simulink model "Copy_of_model_PID"  (R2015a)
settings: Solver=ode4  StartTime=0.0  StopTime=T_sim  FixedStep=0.01  RelTol=1e-3
values from neighbouring files (symbols this model uses):
  D1 = Nastawy(3)    [SzukanieNastaw.m]    (also in wskaznikJakosci.m = params(3))
  h0 = 5    [wskaznikJakosci.m]
  I1 = Nastawy(2)    [SzukanieNastaw.m]    (also in wskaznikJakosci.m = params(2))
  P1 = Nastawy(1)    [SzukanieNastaw.m]    (also in wskaznikJakosci.m = params(1))
  ref = 30    [wskaznikJakosci.m]
undefined symbols (not defined in the file or in its folder): pompaP1, sigbuilder_block, zaworC1, zaworC2, zaworP1
libraries: simulink x1
settings Model: Creator=konra  LastModifiedBy=konra

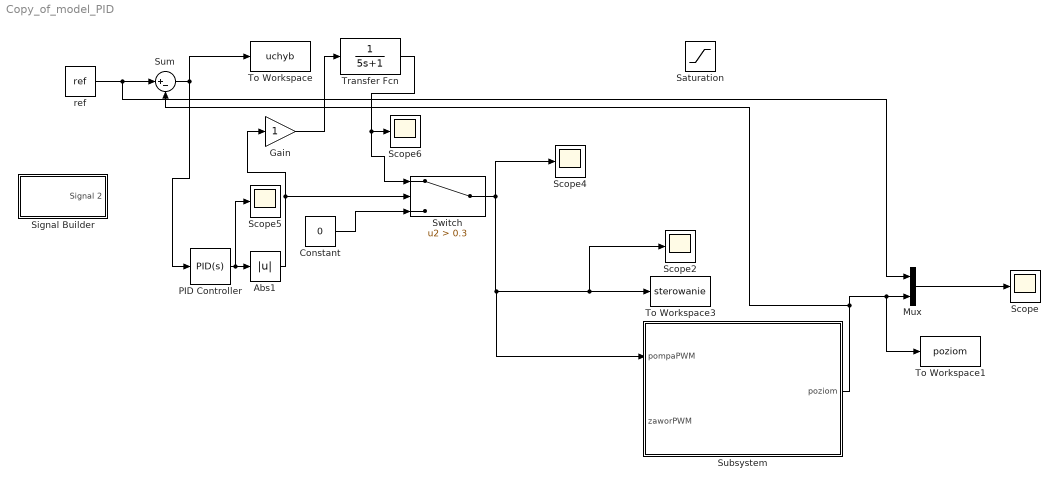
== system Copy_of_model_PID ==
  Abs1 : Abs
  Constant : Constant  Value=0
  Gain : Gain
  Mux : Mux  Inputs=2
  PID Controller : simulink/Continuous/PID Controller  Controller=PID  TimeDomain=Continuous-time  SampleTime=-1  IntegratorMethod=Forward Euler  FilterMethod=Forward Euler  Form=Parallel  UseFilter=on  ControllerParametersSource=internal  P=P1  I=I1  D=D1  N=100  InitialConditionSource=internal  InitialConditionForIntegrator=0  InitialConditionForFilter=0  ExternalReset=none  LimitOutput=on  UpperSaturationLimit=0.8  LowerSaturationLimit=0.3  LinearizeAsGain=on  AntiWindupMode=none  Kb=1  TrackingMode=off  Kt=1  PParamMin=[]  PParamMax=[]  IParamMin=[]  IParamMax=[]  DParamMin=[]  DParamMax=[]  NParamMin=[]  NParamMax=[]  KbParamMin=[]  KbParamMax=[]  KtParamMin=[]  KtParamMax=[]  POutMin=[]  POutMax=[]  IOutMin=[]  IOutMax=[]  DOutMin=[]  DOutMax=[]  NOutMin=[]  NOutMax=[]  KbOutMin=[]  KbOutMax=[]  KtOutMin=[]  KtOutMax=[]  IntegratorOutMin=[]  IntegratorOutMax=[]  FilterOutMin=[]  FilterOutMax=[]  SumOutMin=[]  SumOutMax=[]  SumI1OutMin=[]  SumI1OutMax=[]  SumI2OutMin=[]  SumI2OutMax=[]  SumI3OutMin=[]  SumI3OutMax=[]  SumDOutMin=[]  SumDOutMax=[]  SaturationOutMin=[]  SaturationOutMax=[]  IntegratorContinuousStateAttributes=''  IntegratorStateMustResolveToSignalObject=off  IntegratorRTWStateStorageClass=Auto  FilterContinuousStateAttributes=''  FilterStateMustResolveToSignalObject=off  FilterRTWStateStorageClass=Auto  DifferentiatorICPrevScaledInput=0  DifferentiatorOutMin=[]  DifferentiatorOutMax=[]
  Saturation : Saturate  UpperLimit=0.8  LowerLimit=0.3
  Scope{,2,4..6} (5 alike) : Scope
      Scope settings: YMin=5  YMax=30
      Scope2 settings: SaveName=ScopeData4
      Scope4 settings: YMin=5  YMax=30  SaveName=ScopeData6
      Scope5 settings: YMin=5  YMax=30  SaveName=ScopeData7
      Scope6 settings: YMin=5  YMax=30  SaveName=ScopeData8
  Signal Builder : Subsystem  Tag=STV Subsys  LoadFcn=sigbuilder_block('load');  StartFcn=sigbuilder_block('start');  StopFcn=sigbuilder_block('stop');  ClipboardFcn=sigbuilder_block('clipboard');  mask(Sigbuilder block){}
      mask help: Simulink:masks:SigbuilderBlock_MD
      mask init:
      | if ~strcmp(get_param(bdroot(gcbh),'SimulationStatus'),'stopped') tuvar = sigbuilder_block('maskInit'); end
      settings: CopyFcn=sigbuilder_block('copy');  DeleteFcn=sigbuilder_block('delete');  ModelCloseFcn=sigbuilder_block('modelClose');  PreSaveFcn=sigbuilder_block('preSave');  PauseFcn=sigbuilder_block('pause');  ContinueFcn=sigbuilder_block('continue');  NameChangeFcn=sigbuilder_block('namechange');  OpenFcn=sigbuilder_block('open',[437.6 199.2 550.4 400 ]);  CloseFcn=sigbuilder_block('close');
      mask Display: plot(0, 0, 100, 100,[2, 2, 32, 32, 2], [68, 8, 8, 68, 68],[32, 2], [38, 38], [32, 19, 2],[53, 60, 44], [32, 17, 17, 2],[16, 16, 31, 31]);txt = getActiveGroup(gcbh);text(2, 100, txt,'verticalAlignment', 'top');
  Subsystem : Subsystem
  Sum : Sum  Inputs=|+-
  Switch : Switch  Criteria=u2 > Threshold  Threshold=0.3
  To Workspace : ToWorkspace  VariableName=uchyb  SaveFormat=Structure With Time  SampleTime=-1
  To Workspace1 : ToWorkspace  VariableName=poziom  SaveFormat=Structure With Time  SampleTime=-1
  To Workspace3 : ToWorkspace  VariableName=sterowanie  SaveFormat=Structure With Time  SampleTime=-1
  Transfer Fcn : TransferFcn  Denominator=[5 1]
  ref : Constant  Value=ref
  wires:
  Subsystem/1(poziom) -> To Workspace1/1, Mux/2, Sum/2
  Sum/1 -> PID Controller/1, To Workspace/1
  Constant/1 -> Switch/3
  PID Controller/1 -> Scope5/1, Abs1/1
  Abs1/1 -> Gain/1, Switch/2
  Mux/1 -> Scope/1
  ref/1 -> Mux/1, Sum/1
  Transfer Fcn/1 -> Switch/1, Scope6/1
  Gain/1 -> Transfer Fcn/1
  Switch/1 -> Subsystem/1(pompaPWM), Scope2/1, To Workspace3/1, Scope4/1

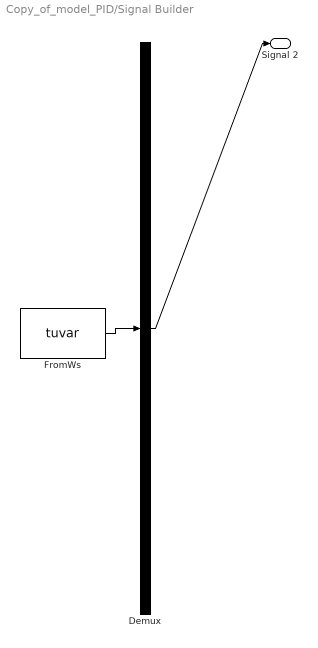
== system Copy_of_model_PID/Signal Builder ==
  Demux : Demux  Tag=STV Demux  Outputs=1
  FromWs : FromWorkspace  Tag=STV FromWs  VariableName=tuvar  SampleTime=0
      SigBuilderData=|
      | common.afterFinalStr = 'Extrapolate'
      | common.sampleTime = 0
      | dataSet.timeRange = [0 300]
      | dataSet.name = 'Group 1'
      | sbobj.Groups.Name = 'Group 1'
      | sbobj.Groups.Signals.Name = 'Signal 2'
      | sbobj.Groups.Signals.XData = [0 80 80 300]
      | sbobj.Groups.Signals.YData = [30 30 5 5]
      | sbobj.Groups.TimeRange = [0 300]
  Signal 2 : Outport  Tag=STV Outport
  wires:
  FromWs/1 -> Demux/1
  Demux/1 -> Signal 2/1

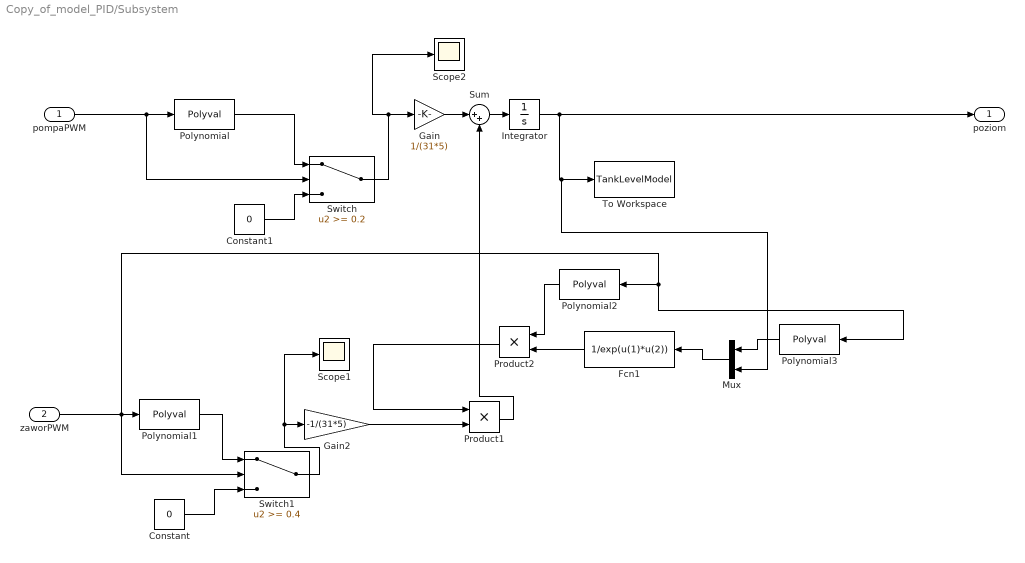
== system Copy_of_model_PID/Subsystem ==
  pompaPWM : Inport
  zaworPWM : Inport  Port=2
  Constant : Constant  Value=0
  Constant1 : Constant  Value=0
  Fcn1 : Fcn  Expr=1/exp(u(1)*u(2))
  Gain : Gain  Gain=1/(31*5)
  Gain2 : Gain  Gain=-1/(31*5)
  Integrator : Integrator  InitialCondition=h0
  Mux : Mux  Inputs=2
  Polynomial : Polyval  Coefs=pompaP1
  Polynomial1 : Polyval  Coefs=zaworP1
  Polynomial2 : Polyval  Coefs=zaworC2
  Polynomial3 : Polyval  Coefs=zaworC1
  Product1 : Product
  Product2 : Product
  Scope1 : Scope
  Scope2 : Scope
      settings: SaveName=ScopeData2
  Sum : Sum  Inputs=|++
  Switch : Switch  Threshold=0.2
  Switch1 : Switch  Threshold=0.4
  To Workspace : ToWorkspace  VariableName=TankLevelModel  SaveFormat=Structure With Time  SampleTime=-1
  poziom : Outport
  wires:
  Switch1/1 -> Scope1/1, Gain2/1
  Polynomial1/1 -> Switch1/1
  Constant/1 -> Switch1/3
  Polynomial/1 -> Switch/1
  Constant1/1 -> Switch/3
  Switch/1 -> Scope2/1, Gain/1
  pompaPWM/1 -> Switch/2, Polynomial/1
  Gain2/1 -> Product1/2
  Product1/1 -> Sum/2
  Product2/1 -> Product1/1
  Integrator/1 -> poziom/1, Mux/2, To Workspace/1
  Fcn1/1 -> Product2/2
  zaworPWM/1 -> Switch1/2, Polynomial1/1, Polynomial3/1, Polynomial2/1
  Polynomial2/1 -> Product2/1
  Mux/1 -> Fcn1/1
  Polynomial3/1 -> Mux/1
  Gain/1 -> Sum/1
  Sum/1 -> Integrator/1
